simulink model "MovementDemonstration"  (R2019b)
settings: Solver=FixedStepAuto  StartTime=0.0  StopTime=inf  FixedStep=0.1  MaxStep=0.01  RelTol=1e-3  EnableMultiTasking=on
libraries: arduinolib x6, simulink x4, arduinowifilib x1
settings Model: SILPILModeSetting=veronly  ExtModeTrigDuration=2  Creator=ioannisgeorgilas  LastModifiedBy=Dave_
settings SolverCC: ZeroCrossAlgorithm=Adaptive
settings OptimizationCC: EnhancedBackFolding=on  PassReuseOutputArgsAs=Individual arguments  ZeroExternalMemoryAtStartup=off  ZeroInternalMemoryAtStartup=off  MaxStackSize=64  OptimizeBlockOrder=speed  DifferentSizesBufferReuse=on  OptimizationCustomize=off  EfficientTunableParamExpr=on
settings DebuggingCC: IgnoredZcDiagnostic=none  MultiTaskRateTransMsg=warning  ParameterTunabilityLossMsg=error
settings HardwareCC: ProdBitPerPointer=32  ProdBitPerSizeT=32  ProdBitPerPtrDiffT=32  ProdLargestAtomicInteger=Long  ProdLargestAtomicFloat=Double  ProdWordSize=32  ProdHWDeviceType=ARM Compatible->ARM Cortex
settings SFSimCC: MATLABDynamicMemAlloc=off  CustomCodeUndefinedFunction=UseInterfaceOnly
settings RTWCC: SystemTargetFile=ert.tlc  HardwareBoard=Arduino MKR1000  TLCOptions=-aInlineSetEventsForThisBaseRateFcn=TLC_FALSE -aSuppressMultiTaskScheduler=TLC_FALSE -aRateBasedStepFcn=1  TemplateMakefile=ert_default_tmf  GenerateReport=on  Toolchain=Arduino ARM  BuildConfiguration=Faster Runs  IncludeHyperlinkInReport=on  LaunchReport=on  GenerateTraceInfo=on  GenerateTraceReport=on  GenerateTraceReportSl=on  GenerateTraceReportSf=on  GenerateTraceReportEml=on
settings CodeAppCC: ForceParamTrailComments=on  IgnoreCustomStorageClasses=off  OperatorAnnotations=on  SimulinkDataObjDesc=on  SFDataObjDesc=on  InsertBlockDesc=on
settings ERTTargetCC: SupportContinuousTime=on  SupportVariableSizeSignals=on  ExtModeStaticAllocSize=8192

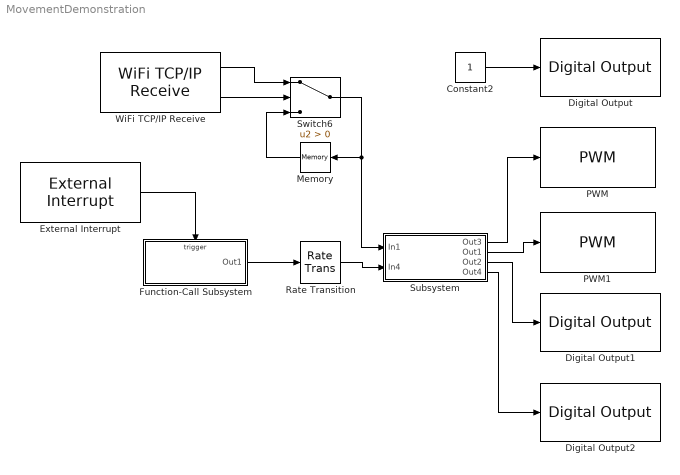
== system MovementDemonstration ==
  Constant2 : Constant
  Digital Output : arduinolib/Digital Output  pinNumber=2  blockPlatform=arduino
  Digital Output1 : arduinolib/Digital Output  pinNumber=0  blockPlatform=arduino
  Digital Output2 : arduinolib/Digital Output  pinNumber=1  blockPlatform=arduino
  External Interrupt : arduinolib/External Interrupt  Pin=16  PullUp=on  Mode=CHANGE  InterruptSimulationInput=off
      settings: SourceProductName=Simulink Support Package for Arduino Hardware  SourceProductBaseCode=ARDUINO
  Function-Call Subsystem : Subsystem  TreatAsAtomicUnit=on
  Memory : Memory
  PWM : arduinolib/PWM  pinNumber=3  EnableInputFrequency=off  InitialFrequency=2000  InitialDutyCycle=0  NotificationType=None  blockPlatform=arduino
  PWM1 : arduinolib/PWM  pinNumber=4  EnableInputFrequency=off  InitialFrequency=2000  InitialDutyCycle=0  NotificationType=None  blockPlatform=arduino
  Rate Transition : RateTransition  Deterministic=off  OutPortSampleTime=0.1
  Subsystem : Subsystem
  Switch6 : Switch  Criteria=u2 > Threshold
  WiFi TCP/IP Receive : arduinowifilib/WiFi TCP//IP Receive  Mode_=Server  serverport=25000  RemoteAddr_=192.168.1.2  RemoteServerPort_=25000  DataType_=uint8  DataSize_=1  SampleTime_=0.1  remoteipoctet1=192  remoteipoctet2=168  remoteipoctet3=1  remoteipoctet4=2  wifiTCPServerIndex=0  wifiTCPClientIndex=0  blockPlatform=ARDUINO  isARMArch=true  SimulateUsing=Code generation  BlockingMode_=off  BlockTimeout_=0.1
      settings: SourceProductName=Simulink Support Package for Arduino Hardware  SourceProductBaseCode=ARDUINO
  wires:
  Constant2/1 -> Digital Output/1
  Function-Call Subsystem/1(Out1) -> Rate Transition/1
  External Interrupt/1 -> Function-Call Subsystem/Trigger
  Subsystem/1(Out3) -> PWM/1
  Rate Transition/1 -> Subsystem/2(In4)
  WiFi TCP/IP Receive/2 -> Switch6/2
  WiFi TCP/IP Receive/1 -> Switch6/1
  Switch6/1 -> Subsystem/1(In1), Memory/1
  Memory/1 -> Switch6/3
  Subsystem/2(Out1) -> PWM1/1
  Subsystem/3(Out2) -> Digital Output1/1
  Subsystem/4(Out4) -> Digital Output2/1

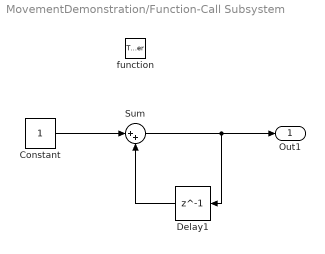
== system MovementDemonstration/Function-Call Subsystem ==
  function : TriggerPort  TriggerType=function-call  VariantControl=Variant
  Constant : Constant
  Delay1 : Delay  DelayLength=1  InitialCondition=0
  Sum : Sum  Inputs=|++  AccumDataTypeStr=double  OutDataTypeStr=double
  Out1 : Outport  OutDataTypeStr=double
  wires:
  Constant/1 -> Sum/1
  Sum/1 -> Delay1/1, Out1/1
  Delay1/1 -> Sum/2

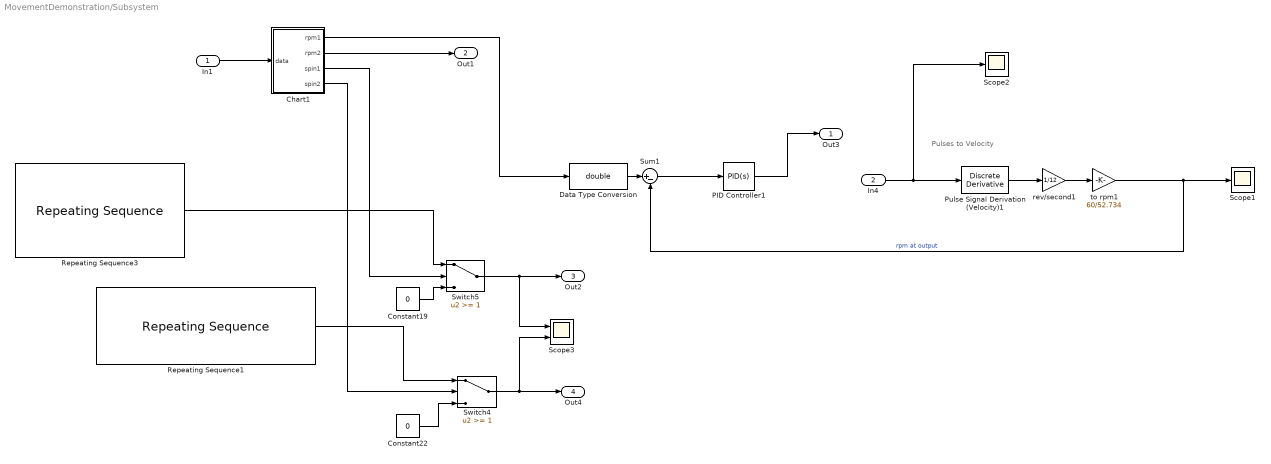
== system MovementDemonstration/Subsystem ==
  note: Pulses to Velocity
  In1 : Inport
  In4 : Inport  Port=2
  Chart1 : Stateflow chart  BlockKeywords=__PRM__SERIALIZED__DATA__:Stateflow Chart,Stateflow Diagram  TreatAsAtomicUnit=on
  Constant19 : Constant  Value=0
  Constant22 : Constant  Value=0
  Data Type Conversion : DataTypeConversion  OutDataTypeStr=double
  PID Controller1 : simulink/Continuous/PID Controller  Controller=PID  Form=Parallel  TimeDomain=Continuous-time  SampleTime=-1  IntegratorMethod=Forward Euler  FilterMethod=Forward Euler  ControllerParametersSource=internal  P=100  I=1  D=0  UseFilter=on  N=100  TunerSelectOption=Transfer Function Based (PID Tuner App)  InitialConditionSource=internal  InitialConditionForIntegrator=0  InitialConditionForFilter=0  DifferentiatorICPrevScaledInput=0  ExternalReset=none  TrackingMode=off  Kt=1  LimitOutput=on  UpperSaturationLimit=255  LowerSaturationLimit=0  LinearizeAsGain=on  AntiWindupMode=clamping  Kb=1  POutMin=[]  POutMax=[]  IOutMin=[]  IOutMax=[]  DOutMin=[]  DOutMax=[]  NOutMin=[]  NOutMax=[]  SumOutMin=[]  SumOutMax=[]  SaturationOutMin=[]  SaturationOutMax=[]  PParamMin=[]  PParamMax=[]  IParamMin=[]  IParamMax=[]  DParamMin=[]  DParamMax=[]  NParamMin=[]  NParamMax=[]  KbParamMin=[]  KbParamMax=[]  KtParamMin=[]  KtParamMax=[]  KbOutMin=[]  KbOutMax=[]  KtOutMin=[]  KtOutMax=[]  IntegratorOutMin=[]  IntegratorOutMax=[]  FilterOutMin=[]  FilterOutMax=[]  SumI1OutMin=[]  SumI1OutMax=[]  SumI2OutMin=[]  SumI2OutMax=[]  SumI3OutMin=[]  SumI3OutMax=[]  SumI4OutMin=[]  SumI4OutMax=[]  SumDOutMin=[]  SumDOutMax=[]  DifferentiatorOutMin=[]  DifferentiatorOutMax=[]  FilterDiffOutCoefMin=[]  FilterDiffOutCoefMax=[]  ReciprocalOutMin=[]  ReciprocalOutMax=[]  SumDenOutMin=[]  SumDenOutMax=[]  SumNumOutMin=[]  SumNumOutMax=[]  DivideOutMin=[]  DivideOutMax=[]  IntegratorContinuousStateAttributes=''  IntegratorStateMustResolveToSignalObject=off  IntegratorRTWStateStorageClass=Auto  FilterContinuousStateAttributes=''  FilterStateMustResolveToSignalObject=off  FilterRTWStateStorageClass=Auto  ParallelPVariant=InternalParameters  IdealPVariant=Disabled  IVariant=InternalParameters  DVariant=InternalParameters  IntegratorVariant=Continuous  SatVariant=Enabled  AWVariant=ContClampingParallel  PCopyVariant=Disabled  TRVariant=Disabled  FdbkBlocksVariant=Forward  IdealPFdbkVariant=Disabled  SatFdbkVariant=Disabled  DerivativeFilterVariant=ContFilter  NVariant=InternalParameters  NCopyVariant=Disabled  FilterICVariant=InternalICsFilter  IntegratorICVariant=InternalICs  ExternalResetVariant=Disabled  TRSumVariant=Passthrough  SumFdbkVariant=Disabled  SumVariant=Sum_PID
  Pulse Signal Derivation (Velocity)1 : simulink/Discrete/Discrete Derivative  gainval=1.0  ICPrevScaledInput=0.0  OutMin=[]  OutMax=[]  OutDataType=fixdt(1, 16)  OutScaling=2^-10  DoSatur=off
  Repeating Sequence1 : simulink/Sources/Repeating Sequence  rep_seq_t=[0 0.25 0.75 1]  rep_seq_y=[1 1 0 0]
  Repeating Sequence3 : simulink/Sources/Repeating Sequence  rep_seq_t=[0 0.25 0.5 0.6 2]  rep_seq_y=[1 1 0.75 0 0]
  Scope1 : Scope
  Scope2 : Scope
  Scope3 : Scope  NumInputPorts=2
  Sum1 : Sum  Inputs=|+-
  Switch4 : Switch  Threshold=1
  Switch5 : Switch  Threshold=1
  rev/second1 : Gain  Gain=1/12
  to rpm1 : Gain  Gain=60/52.734
  Out3 : Outport
  Out1 : Outport  Port=2
  Out2 : Outport  Port=3
  Out4 : Outport  Port=4
  wires:
  Sum1/1 -> PID Controller1/1
  rev/second1/1 -> to rpm1/1
  Data Type Conversion/1 -> Sum1/1
  Pulse Signal Derivation (Velocity)1/1 -> rev/second1/1
  to rpm1/1 -> Scope1/1, Sum1/2  "rpm at output"
  In1/1 -> Chart1/1(data)
  In4/1 -> Scope2/1, Pulse Signal Derivation (Velocity)1/1
  Chart1/2(rpm2) -> Out1/1
  PID Controller1/1 -> Out3/1
  Chart1/1(rpm1) -> Data Type Conversion/1
  Switch4/1 -> Out4/1, Scope3/2
  Switch5/1 -> Out2/1, Scope3/1
  Constant22/1 -> Switch4/3
  Repeating Sequence1/1 -> Switch4/1
  Chart1/3(spin1) -> Switch5/2
  Chart1/4(spin2) -> Switch4/2
  Repeating Sequence3/1 -> Switch5/1
  Constant19/1 -> Switch5/3

== stateflow chart MovementDemonstration/Subsystem/Chart1 ==
  state Start
    entry:
    rpm1=0;
    rpm2=0;
    spin1=0;
    spin2=0;
  state Move
    entry:
    rpm1=20;
    rpm2=0;
    spin1=0;
    spin2=0;
  state Move2
    entry:
    rpm1=0;
    rpm2=20;
    spin1=0;
    spin2=0;
  state Move4
    entry:
    rpm1=0;
    rpm2=0;
    spin1=0;
    spin2=100;
  state Move3
    entry:
    rpm1=0;
    rpm2=0;
    spin1=100;
    spin2=0;
  state Move1
    entry:
    rpm1=0;
    rpm2=0;
    spin1=0;
    spin2=0;
  (default) -> Start
  Move2 -> Start : after(1500,msec)
  Move -> Start : after(1500,msec)
  Start -> Move [order 1] : [data==119]
  Start -> Move2 [order 3] : [data==115]
  Move3 -> Start : after(10000,msec)
  Start -> Move3 [order 4] : [data ==100]
  Start -> Move1 [order 2] : [data==112]
  Move1 -> Start : after(100,msec)
  Move4 -> Start : after(10000,msec)
  Start -> Move4 [order 5] : [data == 97]
  data: data input; rpm1 output; rpm2 output; spin1 output; spin2 output
